simulink model "Sdomain"  (R2023b)
settings: Solver=VariableStepAuto  StartTime=0.0  StopTime=100  RelTol=1e-3
libraries: cstblocks x1
settings Model: Creator=Administrator  LastModifiedBy=Administrator

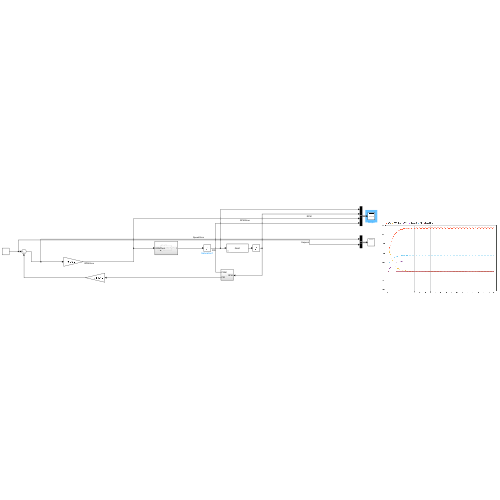
[thumbnail: Simulink's stored preview of the top-level diagram]
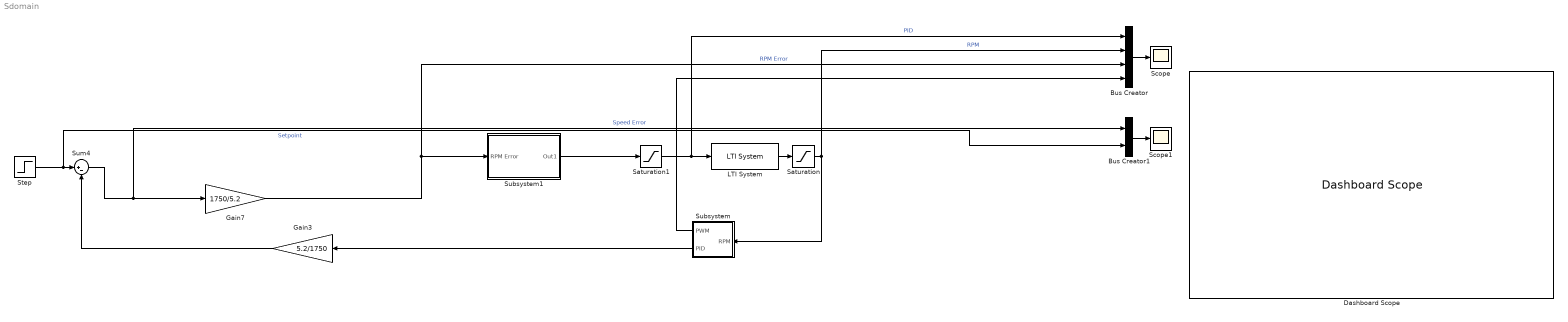
== system Sdomain ==
  Bus Creator : BusCreator  Inputs=4
  Bus Creator1 : BusCreator  Inputs=2
  Dashboard Scope : DashboardScope
  Gain3 : Gain  Gain=5.2/1750
  Gain7 : Gain  Gain=1750/5.2
  LTI System : cstblocks/LTI System  sys=Gest  IC=[]  PadeOrder=0
  Saturation : Saturate  UpperLimit=3600  LowerLimit=900
  Saturation1 : Saturate  UpperLimit=10000  LowerLimit=-1
  Scope : Scope
  Scope1 : Scope
  Step : Step  After=7  SampleTime=0
  Subsystem : Subsystem
  Subsystem1 : Subsystem
  Sum4 : Sum  Inputs=|+-
  wires:
  LTI System/1 -> Saturation/1
  Sum4/1 -> Bus Creator1/1, Gain7/1  "Speed Error"
  Gain3/1 -> Sum4/2
  Step/1 -> Bus Creator1/2, Sum4/1  "Setpoint"
  Saturation/1 -> Subsystem/1(RPM), Bus Creator/2  "RPM"
  Gain7/1 -> Bus Creator/3, Subsystem1/1(RPM Error)  "RPM Error"
  Saturation1/1 -> Bus Creator/1, LTI System/1  "PID"
  Bus Creator/1 -> Scope/1
  Subsystem/1(PWM) -> Bus Creator/4
  Subsystem/2(PID) -> Gain3/1
  Subsystem1/1(Out1) -> Saturation1/1
  Bus Creator1/1 -> Scope1/1

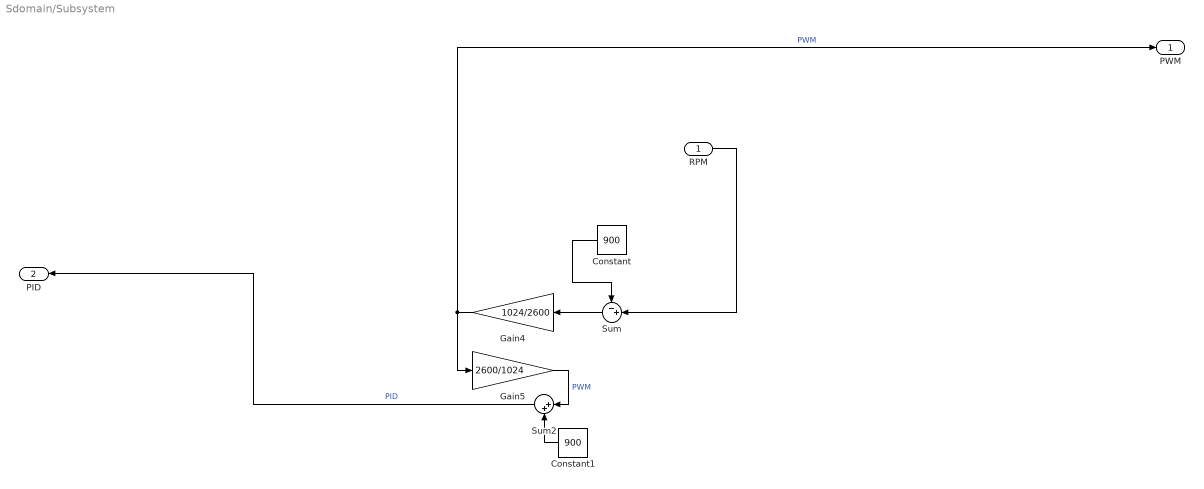
== system Sdomain/Subsystem ==
  RPM : Inport
  Constant : Constant  Value=900
  Constant1 : Constant  Value=900
  Gain4 : Gain  Gain=1024/2600
  Gain5 : Gain  Gain=2600/1024
  Sum : Sum  Inputs=-+|
  Sum2 : Sum  Inputs=|++
  PWM : Outport
  PID : Outport  Port=2
  wires:
  Sum2/1 -> PID/1  "PID"
  Constant/1 -> Sum/1
  Sum/1 -> Gain4/1
  Gain4/1 -> Gain5/1, PWM/1  "PWM"
  Constant1/1 -> Sum2/2
  Gain5/1 -> Sum2/1  "PWM"
  RPM/1 -> Sum/2

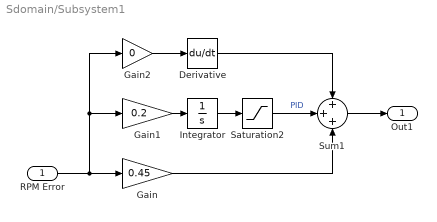
== system Sdomain/Subsystem1 ==
  RPM Error : Inport
  Derivative : Derivative
  Gain : Gain  Gain=0.45
  Gain1 : Gain  Gain=0.2
  Gain2 : Gain  Gain=0
  Integrator : Integrator
  Saturation2 : Saturate  UpperLimit=10000  LowerLimit=0
  Sum1 : Sum  Inputs=+++
  Out1 : Outport
  wires:
  RPM Error/1 -> Gain/1, Gain2/1, Gain1/1
  Gain/1 -> Sum1/3
  Derivative/1 -> Sum1/1
  Integrator/1 -> Saturation2/1
  Saturation2/1 -> Sum1/2  "PID"
  Gain2/1 -> Derivative/1
  Gain1/1 -> Integrator/1
  Sum1/1 -> Out1/1
